simulink model "Equivalency"  (R2018a)
settings: Solver=ode8  StartTime=0.0  StopTime=Ttot  FixedStep=Ts  RelTol=1e-3
values from neighbouring files (symbols this model uses):
  Bench = []    [Equivalency_Script.m]    (also in ShortPulse_Script.m)
  Fn = 60    [Equivalency_Script.m]    (also in FreqAdaptiveFFT_Script.m; FreqAdaptive_Script.m; ShortPulse_Script.m)
  Ts = Ts_control / 60    (= 9.25925925926e-07)    [Equivalency_Script.m]    (also in FreqAdaptiveFFT_Script.m; FreqAdaptive_Script.m; ShortPulse_Script.m)
  Ts_control = 1/(300*Fn)    (= 5.55555555556e-05)    [Equivalency_Script.m]    (also in FreqAdaptiveFFT_Script.m; FreqAdaptive_Script.m; ShortPulse_Script.m)
libraries: DSCdq_Library x16, powerlib x3
settings Model: SimulationMode=accelerator  Creator=daniemot  LastModifiedBy=daniemot
settings SolverCC: AutoInsertRateTranBlk=on
settings DataIOCC: ExternalInput=getinputstruct(WN_50mF_op_snapshot1)  InitialState=getstatestruct(WN_50mF_op_snapshot1)  SaveFinalState=on  SaveFormat=StructureWithTime  SaveOutput=off  SignalLogging=off  DSMLogging=off  SaveTime=off
settings DebuggingCC: ReadBeforeWriteMsg=DisableAll  WriteAfterWriteMsg=DisableAll  WriteAfterReadMsg=DisableAll  MultiTaskDSMMsg=none  UnconnectedInputMsg=none  UnconnectedOutputMsg=none  UnconnectedLineMsg=none
settings ModelReferenceCC: UpdateModelReferenceTargets=IfOutOfDate
settings SFSimCC: SFSimEcho=off

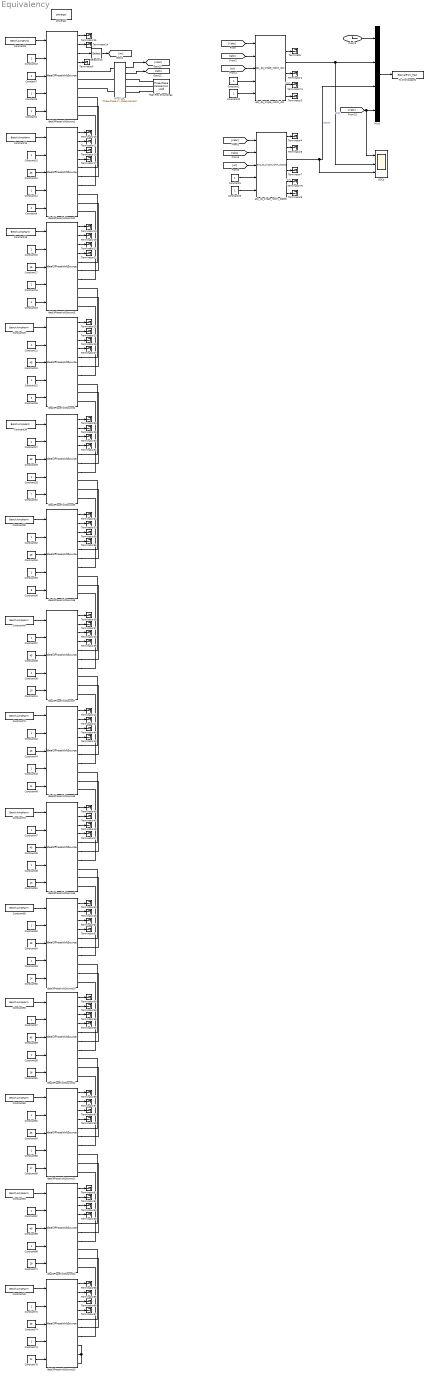
== system Equivalency ==
  Clock3 : Clock
  Constant{1..3,6,10..11,13,15..16,20..23,27..28,32..33,37..38,42..43,47..48,52..53,57..58,62..63,67..68,72..73} (33 alike) : Constant
  Constant{12,17,24,29,34,39,44,49,54,59,64,69,74} (13 alike) : Constant  Value=45
  Constant{14,18,25,30,35,40,45,50,55,60,65,70,75} (13 alike) : Constant  Value=Bench.AmpHarm
  Constant19 : Constant  Value=4
  Constant26 : Constant  Value=5
  Constant31 : Constant  Value=7
  Constant36 : Constant  Value=8
  Constant41 : Constant  Value=10
  Constant46 : Constant  Value=11
  Constant51 : Constant  Value=13
  Constant56 : Constant  Value=14
  Constant61 : Constant  Value=16
  Constant66 : Constant  Value=17
  Constant7 : Constant  Value=0
  Constant71 : Constant  Value=19
  Constant76 : Constant  Value=21
  Constant8 : Constant  Value=Bench.AmpFund
  Constant9 : Constant  Value=2
  "DSCs " : Scope  NumInputPorts=3
  High Res Grounding4 : powerlib/Elements/Three-Phase Parallel RLC Load  LConnTagsString=A|B|C  Configuration=Y (grounded)  NominalVoltage=(1/2^0.5)*3^0.5  Vabc=[1e3 1e3 1e3]  Vabcp=[1e3 1e3 1e3]  NominalFrequency=Fn  UnbalancedPower=off  ActivePower=3/2  InductivePower=0  CapacitivePower=0  Pabc=[10e3 9e3 11e3]  QLabc=[100 90 110]  QCabc=[100 90 110]  Pabcp=[10e3 9e3 11e3]  QLabcp=[100 90 110]  QCabcp=[100 90 110]  Measurements=None  LoadType=constant Z
  Ideal3PhaseVoltSource{1..14} (14 alike) : DSCdq_Library/Ideal3PhaseVoltSource  BaseAmp=1  fn=Fn
  Mux1 : Mux
  Selector10 : Selector  InputPortWidth=3  IndexOptions=Index vector (dialog)  Indices=[1]  OutputSizes=1
  Terminator{,1,3..7,9,11,16..68,74..75} (64 alike) : Terminator
  To Workspace1 : ToWorkspace  VariableName=Equivalency_Raw  SampleTime=Ts_control
      settings: Save2DSignal=2-D array (concatenate along first dimension)
  WT3_LSC : powerlib/Measurements/Three-Phase V-I Measurement  VoltageMeasurement=phase-to-ground  SetLabelV=off  LabelV=vgrid  Vpu=off  VpuLL=off  CurrentMeasurement=yes  SetLabelI=off  LabelI=igrid  Ipu=off  Pbase=sn  Vbase=uab  OutputType=Complex  PhasorSimulation=off  PSBequivalent=0
  abc_dq_single_notch_dqDSC : DSCdq_Library/abc_dq_single_notch_dqDSC  Ts=Ts_control  fn=Fn  fmin=0.8*Fn  zeta=zeta
  abc_dq_single_notch_dsc : DSCdq_Library/abc_dq_single_notch_dsc  Ts=Ts_control  fn=Fn  fmin=0.8*Fn  zeta=zeta
  powergui : powerlib/powergui  Priority=1  SimulationMode=Discrete  SampleTime=Ts  frequency=60  Iterations=50  frequencyindice=0  Pbase=100e6  ErrMax=1e-4  UnitsV=kV  UnitsW=MW  buscounter=0  FunctionMessages=off  echomessages=off  EnableUseOfTLC=off  CurrentSourceSwitches=off  DisableSnubberDevices=off  DisableRonSwitches=off  DisableVfSwitches=off  DisplayEquations=off  SolverType=Tustin/Backward Euler (TBE)  Interpol=off  ExternalGateDelay=off  methode=off  Ts=100  x0status=blocks  SPID=off  SwTol=0  HookPort=off  RestoreLinks=warning  ResistiveCurrentMeasurement=off  Frange=[60:1:1600]  Ylog=on  Xlog=on  ShowGrid=on  save=off  variable=ZData  structure=0  ZoomFFT=off  StartTime=0.0  cycles=1  DisplayStyle=1  fundamental=60  FreqAxis=off  MaxFrequency=1000  frequencyindicesteady=1  RmsSteady=1  display=off
  wires:
  Constant6/1 -> Ideal3PhaseVoltSource1/4
  Constant7/1 -> Ideal3PhaseVoltSource1/3
  Constant13/1 -> Ideal3PhaseVoltSource1/2
  Ideal3PhaseVoltSource1/3 -> Selector10/1
  Ideal3PhaseVoltSource1/2 -> Terminator24/1
  Ideal3PhaseVoltSource1/1 -> Terminator25/1
  WT3_LSC/1 -> [Vabc]
  Ideal3PhaseVoltSource1/4 -> Terminator5/1
  Clock3/1 -> Mux1/1
  Mux1/1 -> To Workspace1/1
  Constant8/1 -> Ideal3PhaseVoltSource1/1
  Constant20/1 -> abc_dq_single_notch_dsc/5
  Constant1/1 -> Ideal3PhaseVoltSource1/5
  Constant23/1 -> abc_dq_single_notch_dqDSC/5
  Selector10/1 -> [wt]
  [Vabc] -> abc_dq_single_notch_dsc/1
  [Vabc] -> abc_dq_single_notch_dqDSC/1
  [Iabc] -> abc_dq_single_notch_dsc/2
  [Iabc] -> abc_dq_single_notch_dqDSC/2
  [wt] -> abc_dq_single_notch_dsc/3
  [wt] -> abc_dq_single_notch_dqDSC/3
  Constant2/1 -> abc_dq_single_notch_dsc/4
  Constant3/1 -> abc_dq_single_notch_dqDSC/4
  abc_dq_single_notch_dsc/2 -> Terminator/1
  abc_dq_single_notch_dsc/4 -> Terminator1/1
  abc_dq_single_notch_dsc/6 -> Terminator3/1
  abc_dq_single_notch_dqDSC/1 -> Terminator4/1
  abc_dq_single_notch_dqDSC/2 -> Terminator6/1
  abc_dq_single_notch_dqDSC/4 -> Terminator7/1
  abc_dq_single_notch_dqDSC/6 -> Terminator9/1
  WT3_LSC/2 -> [Iabc]
  Ideal3PhaseVoltSource2/2 -> Terminator11/1
  Constant11/1 -> Ideal3PhaseVoltSource2/4
  Constant9/1 -> Ideal3PhaseVoltSource2/5
  Constant12/1 -> Ideal3PhaseVoltSource2/3
  Ideal3PhaseVoltSource2/1 -> Terminator16/1
  Ideal3PhaseVoltSource2/4 -> Terminator17/1
  Constant10/1 -> Ideal3PhaseVoltSource2/2
  Constant14/1 -> Ideal3PhaseVoltSource2/1
  Ideal3PhaseVoltSource2/3 -> Terminator18/1
  Constant15/1 -> Ideal3PhaseVoltSource3/2
  Constant17/1 -> Ideal3PhaseVoltSource3/3
  Ideal3PhaseVoltSource3/1 -> Terminator20/1
  Constant19/1 -> Ideal3PhaseVoltSource3/5
  Ideal3PhaseVoltSource3/4 -> Terminator21/1
  Ideal3PhaseVoltSource3/2 -> Terminator19/1
  Constant18/1 -> Ideal3PhaseVoltSource3/1
  Constant16/1 -> Ideal3PhaseVoltSource3/4
  Ideal3PhaseVoltSource3/3 -> Terminator22/1
  Constant22/1 -> Ideal3PhaseVoltSource4/4
  Ideal3PhaseVoltSource4/2 -> Terminator23/1
  Constant25/1 -> Ideal3PhaseVoltSource4/1
  Constant21/1 -> Ideal3PhaseVoltSource4/2
  Ideal3PhaseVoltSource4/1 -> Terminator26/1
  Ideal3PhaseVoltSource4/3 -> Terminator28/1
  Constant26/1 -> Ideal3PhaseVoltSource4/5
  Constant24/1 -> Ideal3PhaseVoltSource4/3
  Ideal3PhaseVoltSource4/4 -> Terminator27/1
  Ideal3PhaseVoltSource5/3 -> Terminator32/1
  Constant27/1 -> Ideal3PhaseVoltSource5/2
  Ideal3PhaseVoltSource5/4 -> Terminator31/1
  Ideal3PhaseVoltSource5/1 -> Terminator30/1
  Constant30/1 -> Ideal3PhaseVoltSource5/1
  Constant29/1 -> Ideal3PhaseVoltSource5/3
  Ideal3PhaseVoltSource5/2 -> Terminator29/1
  Constant28/1 -> Ideal3PhaseVoltSource5/4
  Constant31/1 -> Ideal3PhaseVoltSource5/5
  Constant36/1 -> Ideal3PhaseVoltSource6/5
  Constant34/1 -> Ideal3PhaseVoltSource6/3
  Ideal3PhaseVoltSource6/2 -> Terminator33/1
  Ideal3PhaseVoltSource6/1 -> Terminator34/1
  Constant35/1 -> Ideal3PhaseVoltSource6/1
  Constant33/1 -> Ideal3PhaseVoltSource6/4
  Ideal3PhaseVoltSource6/4 -> Terminator35/1
  Ideal3PhaseVoltSource6/3 -> Terminator36/1
  Constant32/1 -> Ideal3PhaseVoltSource6/2
  Constant42/1 -> Ideal3PhaseVoltSource8/2
  Ideal3PhaseVoltSource8/3 -> Terminator44/1
  Ideal3PhaseVoltSource8/4 -> Terminator43/1
  Constant43/1 -> Ideal3PhaseVoltSource8/4
  Constant75/1 -> Ideal3PhaseVoltSource8/1
  Ideal3PhaseVoltSource8/1 -> Terminator42/1
  Constant44/1 -> Ideal3PhaseVoltSource8/3
  Ideal3PhaseVoltSource8/2 -> Terminator41/1
  Constant46/1 -> Ideal3PhaseVoltSource8/5
  Constant41/1 -> Ideal3PhaseVoltSource7/5
  Constant39/1 -> Ideal3PhaseVoltSource7/3
  Ideal3PhaseVoltSource7/2 -> Terminator37/1
  Ideal3PhaseVoltSource7/1 -> Terminator38/1
  Constant40/1 -> Ideal3PhaseVoltSource7/1
  Constant38/1 -> Ideal3PhaseVoltSource7/4
  Ideal3PhaseVoltSource7/4 -> Terminator39/1
  Ideal3PhaseVoltSource7/3 -> Terminator40/1
  Constant37/1 -> Ideal3PhaseVoltSource7/2
  Constant47/1 -> Ideal3PhaseVoltSource9/2
  Constant48/1 -> Ideal3PhaseVoltSource9/4
  Ideal3PhaseVoltSource9/4 -> Terminator47/1
  Ideal3PhaseVoltSource9/3 -> Terminator48/1
  Ideal3PhaseVoltSource9/1 -> Terminator46/1
  Constant70/1 -> Ideal3PhaseVoltSource9/1
  Ideal3PhaseVoltSource9/2 -> Terminator45/1
  Constant49/1 -> Ideal3PhaseVoltSource9/3
  Constant51/1 -> Ideal3PhaseVoltSource9/5
  Constant54/1 -> Ideal3PhaseVoltSource10/3
  Constant53/1 -> Ideal3PhaseVoltSource10/4
  Constant65/1 -> Ideal3PhaseVoltSource10/1
  Ideal3PhaseVoltSource10/2 -> Terminator49/1
  Ideal3PhaseVoltSource10/3 -> Terminator52/1
  Ideal3PhaseVoltSource10/1 -> Terminator50/1
  Constant52/1 -> Ideal3PhaseVoltSource10/2
  Ideal3PhaseVoltSource10/4 -> Terminator51/1
  Constant56/1 -> Ideal3PhaseVoltSource10/5
  Constant66/1 -> Ideal3PhaseVoltSource11/5
  Constant62/1 -> Ideal3PhaseVoltSource11/2
  Ideal3PhaseVoltSource11/4 -> Terminator59/1
  Ideal3PhaseVoltSource11/2 -> Terminator57/1
  Ideal3PhaseVoltSource11/3 -> Terminator60/1
  Ideal3PhaseVoltSource11/1 -> Terminator58/1
  Constant61/1 -> Ideal3PhaseVoltSource12/5
  Constant63/1 -> Ideal3PhaseVoltSource11/4
  Constant64/1 -> Ideal3PhaseVoltSource11/3
  Constant55/1 -> Ideal3PhaseVoltSource12/1
  Constant59/1 -> Ideal3PhaseVoltSource12/3
  Ideal3PhaseVoltSource12/4 -> Terminator55/1
  Constant58/1 -> Ideal3PhaseVoltSource12/4
  Ideal3PhaseVoltSource12/3 -> Terminator56/1
  Ideal3PhaseVoltSource12/1 -> Terminator54/1
  Constant60/1 -> Ideal3PhaseVoltSource11/1
  Constant57/1 -> Ideal3PhaseVoltSource12/2
  Ideal3PhaseVoltSource12/2 -> Terminator53/1
  Constant67/1 -> Ideal3PhaseVoltSource14/2
  Constant45/1 -> Ideal3PhaseVoltSource13/1
  Ideal3PhaseVoltSource14/2 -> Terminator61/1
  Constant68/1 -> Ideal3PhaseVoltSource14/4
  Ideal3PhaseVoltSource14/4 -> Terminator63/1
  Constant69/1 -> Ideal3PhaseVoltSource14/3
  Constant50/1 -> Ideal3PhaseVoltSource14/1
  Constant74/1 -> Ideal3PhaseVoltSource13/3
  Ideal3PhaseVoltSource14/1 -> Terminator62/1
  Ideal3PhaseVoltSource14/3 -> Terminator64/1
  Constant73/1 -> Ideal3PhaseVoltSource13/4
  Ideal3PhaseVoltSource13/4 -> Terminator67/1
  Constant71/1 -> Ideal3PhaseVoltSource14/5
  Ideal3PhaseVoltSource13/1 -> Terminator66/1
  Constant72/1 -> Ideal3PhaseVoltSource13/2
  Ideal3PhaseVoltSource13/3 -> Terminator68/1
  Constant76/1 -> Ideal3PhaseVoltSource13/5
  Ideal3PhaseVoltSource13/2 -> Terminator65/1
  abc_dq_single_notch_dsc/5 -> Terminator74/1  "Notch"
  abc_dq_single_notch_dqDSC/5 -> Terminator75/1  "DSC"
  abc_dq_single_notch_dsc/3 -> "DSCs "/2, Mux1/2  "DSC"
  abc_dq_single_notch_dqDSC/3 -> "DSCs "/3, Mux1/3  "DSCdq"
  [Vabc] -> "DSCs "/1, Mux1/4
  connections:
  WT3_LSC/LConn1 -- Ideal3PhaseVoltSource1/RConn1
  WT3_LSC/LConn3 -- Ideal3PhaseVoltSource1/RConn3
  WT3_LSC/LConn2 -- Ideal3PhaseVoltSource1/RConn2
  High Res Grounding4/LConn1 -- WT3_LSC/RConn1
  High Res Grounding4/LConn2 -- WT3_LSC/RConn2
  High Res Grounding4/LConn3 -- WT3_LSC/RConn3
  Ideal3PhaseVoltSource13/RConn4 -- Ideal3PhaseVoltSource13/RConn5 -- Ideal3PhaseVoltSource13/RConn6
  Ideal3PhaseVoltSource13/RConn3 -- Ideal3PhaseVoltSource14/RConn6
  Ideal3PhaseVoltSource13/RConn2 -- Ideal3PhaseVoltSource14/RConn5
  Ideal3PhaseVoltSource13/RConn1 -- Ideal3PhaseVoltSource14/RConn4
  Ideal3PhaseVoltSource14/RConn3 -- Ideal3PhaseVoltSource11/RConn6
  Ideal3PhaseVoltSource14/RConn2 -- Ideal3PhaseVoltSource11/RConn5
  Ideal3PhaseVoltSource14/RConn1 -- Ideal3PhaseVoltSource11/RConn4
  Ideal3PhaseVoltSource11/RConn3 -- Ideal3PhaseVoltSource12/RConn6
  Ideal3PhaseVoltSource11/RConn2 -- Ideal3PhaseVoltSource12/RConn5
  Ideal3PhaseVoltSource11/RConn1 -- Ideal3PhaseVoltSource12/RConn4
  Ideal3PhaseVoltSource12/RConn3 -- Ideal3PhaseVoltSource10/RConn6
  Ideal3PhaseVoltSource12/RConn2 -- Ideal3PhaseVoltSource10/RConn5
  Ideal3PhaseVoltSource12/RConn1 -- Ideal3PhaseVoltSource10/RConn4
  Ideal3PhaseVoltSource10/RConn3 -- Ideal3PhaseVoltSource9/RConn6
  Ideal3PhaseVoltSource10/RConn2 -- Ideal3PhaseVoltSource9/RConn5
  Ideal3PhaseVoltSource10/RConn1 -- Ideal3PhaseVoltSource9/RConn4
  Ideal3PhaseVoltSource9/RConn3 -- Ideal3PhaseVoltSource8/RConn6
  Ideal3PhaseVoltSource9/RConn2 -- Ideal3PhaseVoltSource8/RConn5
  Ideal3PhaseVoltSource9/RConn1 -- Ideal3PhaseVoltSource8/RConn4
  Ideal3PhaseVoltSource8/RConn3 -- Ideal3PhaseVoltSource7/RConn6
  Ideal3PhaseVoltSource8/RConn2 -- Ideal3PhaseVoltSource7/RConn5
  Ideal3PhaseVoltSource8/RConn1 -- Ideal3PhaseVoltSource7/RConn4
  Ideal3PhaseVoltSource7/RConn3 -- Ideal3PhaseVoltSource6/RConn6
  Ideal3PhaseVoltSource7/RConn2 -- Ideal3PhaseVoltSource6/RConn5
  Ideal3PhaseVoltSource7/RConn1 -- Ideal3PhaseVoltSource6/RConn4
  Ideal3PhaseVoltSource6/RConn3 -- Ideal3PhaseVoltSource5/RConn6
  Ideal3PhaseVoltSource6/RConn2 -- Ideal3PhaseVoltSource5/RConn5
  Ideal3PhaseVoltSource6/RConn1 -- Ideal3PhaseVoltSource5/RConn4
  Ideal3PhaseVoltSource5/RConn3 -- Ideal3PhaseVoltSource4/RConn6
  Ideal3PhaseVoltSource5/RConn2 -- Ideal3PhaseVoltSource4/RConn5
  Ideal3PhaseVoltSource5/RConn1 -- Ideal3PhaseVoltSource4/RConn4
  Ideal3PhaseVoltSource4/RConn3 -- Ideal3PhaseVoltSource3/RConn6
  Ideal3PhaseVoltSource4/RConn2 -- Ideal3PhaseVoltSource3/RConn5
  Ideal3PhaseVoltSource4/RConn1 -- Ideal3PhaseVoltSource3/RConn4
  Ideal3PhaseVoltSource3/RConn3 -- Ideal3PhaseVoltSource2/RConn6
  Ideal3PhaseVoltSource3/RConn2 -- Ideal3PhaseVoltSource2/RConn5
  Ideal3PhaseVoltSource3/RConn1 -- Ideal3PhaseVoltSource2/RConn4
  Ideal3PhaseVoltSource2/RConn3 -- Ideal3PhaseVoltSource1/RConn6
  Ideal3PhaseVoltSource2/RConn2 -- Ideal3PhaseVoltSource1/RConn5
  Ideal3PhaseVoltSource2/RConn1 -- Ideal3PhaseVoltSource1/RConn4
